simulink model "tres_dummy_aperiodic"  (Simulink 8.3)
settings: Solver=VariableStepDiscrete  StartTime=0.0  StopTime=65  RelTol=1e-3
libraries: tres_simulink_blockset x4
settings Model: Creator=matteo  LastModifiedBy=matteo
settings OptimizationCC: ExpressionDepthLimit=2147483647
settings DebuggingCC: FcnCallInpInsideContextMsg=EnableAllAsWarning
settings GRTTargetCC: CombineOutputUpdateFcns=on  GRTInterface=off

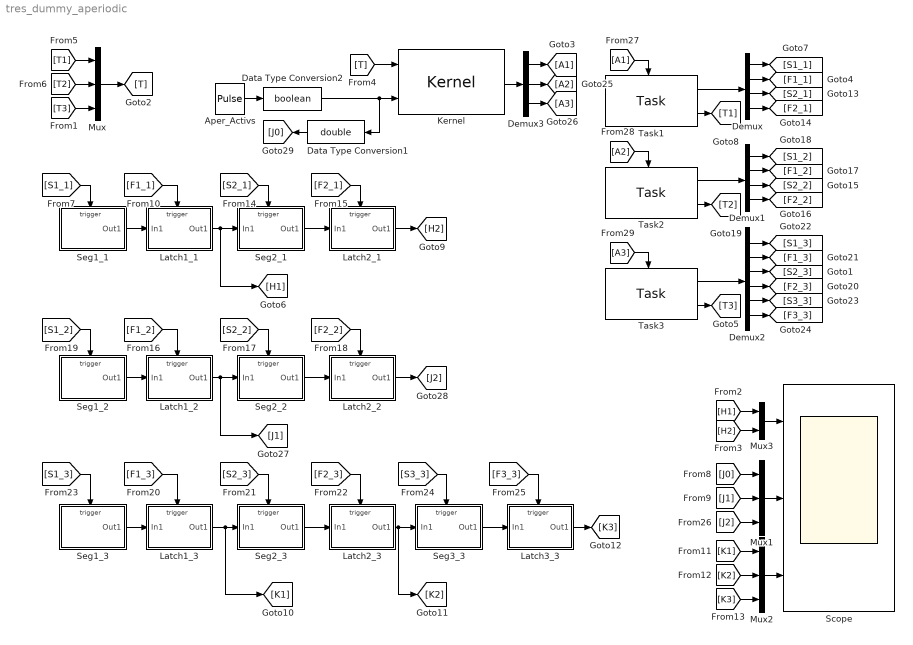
== system tres_dummy_aperiodic ==
  Aper_Activs : DiscretePulseGenerator  PulseType=Time based  Period=16  PulseWidth=100/16  PhaseDelay=16
  Data Type Conversion1 : DataTypeConversion  OutDataTypeStr=double
  Data Type Conversion2 : DataTypeConversion  OutDataTypeStr=boolean
  Demux : Demux
  Demux1 : Demux
  Demux2 : Demux  Outputs=6
  Demux3 : Demux  Outputs=3
  Kernel : tres_simulink_blockset/Kernel  taskset_descr_name=task_set_descr  scheduling_policy=DEADLINE_MONOTONIC  dead_miss_rule=Continue  time_res=Milli_Seconds  core_num=1  under_engine=RTSIM
  Latch1_1 : Subsystem  TreatAsAtomicUnit=on
  Latch1_2 : Subsystem  TreatAsAtomicUnit=on
  Latch1_3 : Subsystem  TreatAsAtomicUnit=on
  Latch2_1 : Subsystem  TreatAsAtomicUnit=on
  Latch2_2 : Subsystem  TreatAsAtomicUnit=on
  Latch2_3 : Subsystem  TreatAsAtomicUnit=on
  Latch3_3 : Subsystem  TreatAsAtomicUnit=on
  Mux : Mux  Inputs=3
  Mux1 : Mux  Inputs=3
  Mux2 : Mux  Inputs=3
  Mux3 : Mux  Inputs=2
  Scope : Scope  NumInputPorts=3
      settings: YMin=-5~-5~-5  YMax=5~5~5
  Seg1_1 : Subsystem  TreatAsAtomicUnit=on
  Seg1_2 : Subsystem  TreatAsAtomicUnit=on
  Seg1_3 : Subsystem  TreatAsAtomicUnit=on
  Seg2_1 : Subsystem  TreatAsAtomicUnit=on
  Seg2_2 : Subsystem  TreatAsAtomicUnit=on
  Seg2_3 : Subsystem  TreatAsAtomicUnit=on
  Seg3_3 : Subsystem  TreatAsAtomicUnit=on
  Task1 : tres_simulink_blockset/Task  conf_name=t1_instrs
  Task2 : tres_simulink_blockset/Task  conf_name=t2_instrs
  Task3 : tres_simulink_blockset/Task  conf_name=t3_instrs
  wires:
  [T] -> Kernel/1
  [T1] -> Mux/1
  [T2] -> Mux/2
  Mux/1 -> [T]
  Task3/2 -> [T3]
  Task1/2 -> [T1]
  Seg1_1/1(Out1) -> Latch1_1/1(In1)
  Latch1_1/1(Out1) -> Seg2_1/1(In1), [H1]
  Seg2_1/1(Out1) -> Latch2_1/1(In1)
  Latch2_1/1(Out1) -> [H2]
  Seg1_3/1(Out1) -> Latch1_3/1(In1)
  Seg2_3/1(Out1) -> Latch2_3/1(In1)
  Latch2_3/1(Out1) -> [K2], Seg3_3/1(In1)
  [K1] -> Mux2/1
  [K2] -> Mux2/2
  Latch1_3/1(Out1) -> [K1], Seg2_3/1(In1)
  Seg3_3/1(Out1) -> Latch3_3/1(In1)
  Latch3_3/1(Out1) -> [K3]
  [K3] -> Mux2/3
  [T3] -> Mux/3
  Task1/1 -> Demux/1
  Demux/1 -> [S1_1]
  Demux/2 -> [F1_1]
  Demux/3 -> [S2_1]
  Demux/4 -> [F2_1]
  Task2/2 -> [T2]
  Task2/1 -> Demux1/1
  Demux1/1 -> [S1_2]
  Demux1/2 -> [F1_2]
  Demux1/3 -> [S2_2]
  Demux1/4 -> [F2_2]
  Demux2/1 -> [S1_3]
  Demux2/2 -> [F1_3]
  Demux2/3 -> [S2_3]
  Demux2/4 -> [F2_3]
  Demux2/5 -> [S3_3]
  Demux2/6 -> [F3_3]
  Task3/1 -> Demux2/1
  Demux3/1 -> [A1]
  Demux3/2 -> [A2]
  Demux3/3 -> [A3]
  Kernel/1 -> Demux3/1
  Seg1_2/1(Out1) -> Latch1_2/1(In1)
  Latch1_2/1(Out1) -> Seg2_2/1(In1), [J1]
  Seg2_2/1(Out1) -> Latch2_2/1(In1)
  Latch2_2/1(Out1) -> [J2]
  [H1] -> Mux3/1
  [H2] -> Mux3/2
  Mux3/1 -> Scope/1
  Mux2/1 -> Scope/3
  [S1_1] -> Seg1_1/Trigger
  [F1_1] -> Latch1_1/Trigger
  [S2_1] -> Seg2_1/Trigger
  [F2_1] -> Latch2_1/Trigger
  [S1_2] -> Seg1_2/Trigger
  [F1_2] -> Latch1_2/Trigger
  [S2_2] -> Seg2_2/Trigger
  [F2_2] -> Latch2_2/Trigger
  [S1_3] -> Seg1_3/Trigger
  [F1_3] -> Latch1_3/Trigger
  [S2_3] -> Seg2_3/Trigger
  [F2_3] -> Latch2_3/Trigger
  [S3_3] -> Seg3_3/Trigger
  [F3_3] -> Latch3_3/Trigger
  [J0] -> Mux1/1
  [J1] -> Mux1/2
  [J2] -> Mux1/3
  Mux1/1 -> Scope/2
  [A1] -> Task1/Trigger
  [A2] -> Task2/Trigger
  [A3] -> Task3/Trigger
  Aper_Activs/1 -> Data Type Conversion2/1
  Data Type Conversion2/1 -> Kernel/2, Data Type Conversion1/1
  Data Type Conversion1/1 -> [J0]

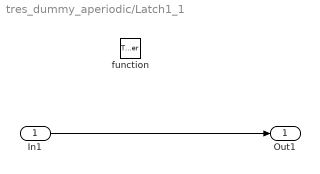
== system tres_dummy_aperiodic/Latch1_1 ==
  In1 : Inport
  function : TriggerPort  TriggerType=function-call
  Out1 : Outport
  wires:
  In1/1 -> Out1/1

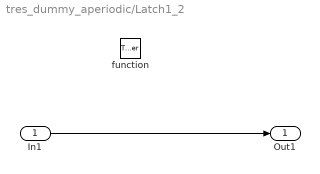
== system tres_dummy_aperiodic/Latch1_2 ==
  In1 : Inport
  function : TriggerPort  TriggerType=function-call
  Out1 : Outport
  wires:
  In1/1 -> Out1/1

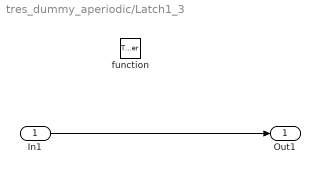
== system tres_dummy_aperiodic/Latch1_3 ==
  In1 : Inport
  function : TriggerPort  TriggerType=function-call
  Out1 : Outport
  wires:
  In1/1 -> Out1/1

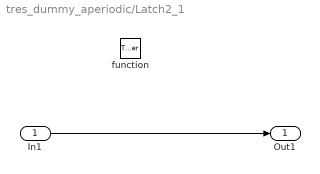
== system tres_dummy_aperiodic/Latch2_1 ==
  In1 : Inport
  function : TriggerPort  TriggerType=function-call
  Out1 : Outport
  wires:
  In1/1 -> Out1/1

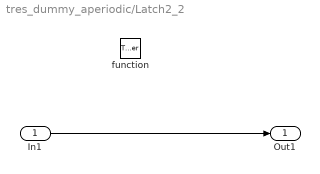
== system tres_dummy_aperiodic/Latch2_2 ==
  In1 : Inport
  function : TriggerPort  TriggerType=function-call
  Out1 : Outport
  wires:
  In1/1 -> Out1/1

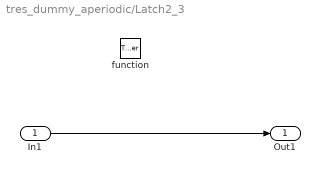
== system tres_dummy_aperiodic/Latch2_3 ==
  In1 : Inport
  function : TriggerPort  TriggerType=function-call
  Out1 : Outport
  wires:
  In1/1 -> Out1/1

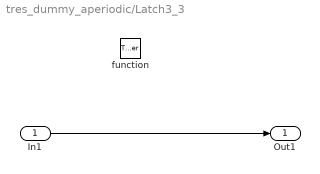
== system tres_dummy_aperiodic/Latch3_3 ==
  In1 : Inport
  function : TriggerPort  TriggerType=function-call
  Out1 : Outport
  wires:
  In1/1 -> Out1/1

== system tres_dummy_aperiodic/Seg1_1 ==
  function : TriggerPort  TriggerType=function-call
  Digital Clock : DigitalClock  SampleTime=-1
  Out1 : Outport
  wires:
  Digital Clock/1 -> Out1/1

== system tres_dummy_aperiodic/Seg1_2 ==
  function : TriggerPort  TriggerType=function-call
  Digital Clock : DigitalClock  SampleTime=-1
  Out1 : Outport
  wires:
  Digital Clock/1 -> Out1/1

== system tres_dummy_aperiodic/Seg1_3 ==
  function : TriggerPort  TriggerType=function-call
  Digital Clock : DigitalClock  SampleTime=-1
  Out1 : Outport
  wires:
  Digital Clock/1 -> Out1/1

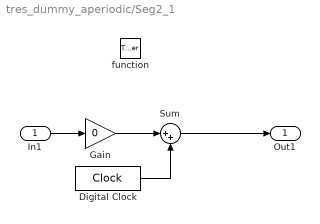
== system tres_dummy_aperiodic/Seg2_1 ==
  In1 : Inport
  function : TriggerPort  TriggerType=function-call
  Digital Clock : DigitalClock  SampleTime=-1
  Gain : Gain  Gain=0
  Sum : Sum  Inputs=|++
  Out1 : Outport
  wires:
  Sum/1 -> Out1/1
  Digital Clock/1 -> Sum/2
  In1/1 -> Gain/1
  Gain/1 -> Sum/1

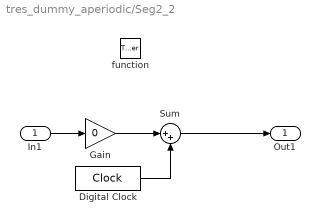
== system tres_dummy_aperiodic/Seg2_2 ==
  In1 : Inport
  function : TriggerPort  TriggerType=function-call
  Digital Clock : DigitalClock  SampleTime=-1
  Gain : Gain  Gain=0
  Sum : Sum  Inputs=|++
  Out1 : Outport
  wires:
  Sum/1 -> Out1/1
  Digital Clock/1 -> Sum/2
  In1/1 -> Gain/1
  Gain/1 -> Sum/1

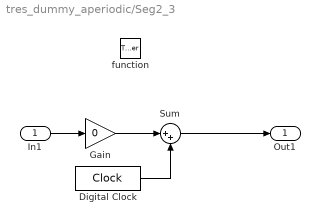
== system tres_dummy_aperiodic/Seg2_3 ==
  In1 : Inport
  function : TriggerPort  TriggerType=function-call
  Digital Clock : DigitalClock  SampleTime=-1
  Gain : Gain  Gain=0
  Sum : Sum  Inputs=|++
  Out1 : Outport
  wires:
  Sum/1 -> Out1/1
  Digital Clock/1 -> Sum/2
  In1/1 -> Gain/1
  Gain/1 -> Sum/1

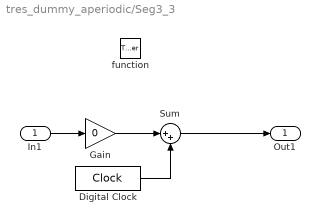
== system tres_dummy_aperiodic/Seg3_3 ==
  In1 : Inport
  function : TriggerPort  TriggerType=function-call
  Digital Clock : DigitalClock  SampleTime=-1
  Gain : Gain  Gain=0
  Sum : Sum  Inputs=|++
  Out1 : Outport
  wires:
  Sum/1 -> Out1/1
  Digital Clock/1 -> Sum/2
  In1/1 -> Gain/1
  Gain/1 -> Sum/1
